simulink model "trenl"  (Simulink 8.8)
settings: Solver=ode45  StartTime=0.0  StopTime=10.0  RelTol=1e-3  EnableMultiTasking=on
values from neighbouring files (symbols this model uses):
  NP = a    [l_2.m]
  R = b    [l_2.m]
  to = randseed    [l_2.m]
  Ts = 0.001    [l_2.m]
libraries: commanapbnd3 x2
settings Model: SuppressorTable=22 serialization::archive 11 0 3 0 0 0 0 0  Creator=MichaelK  LastModifiedBy=tandav
settings DataIOCC: SaveFormat=Dataset  SignalLoggingSaveFormat=Dataset
settings DebuggingCC: UnderspecifiedInitializationDetection=Simplified  MergeDetectMultiDrivingBlocksExec=error  FcnCallInpInsideContextMsg=error  AllowSymbolicDim=off  StateNameClashWarn=none
settings HardwareCC: ProdBitPerPointer=64  ProdBitPerSizeT=64  ProdBitPerPtrDiffT=64  ProdLargestAtomicFloat=Float  ProdIntDivRoundTo=Zero  ProdEndianess=LittleEndian  ProdWordSize=64  ProdHWDeviceType=Intel->x86-64 (Windows64)
settings GRTTargetCC: GeneratePreprocessorConditionals=Use local settings  CombineOutputUpdateFcns=on  GRTInterface=off

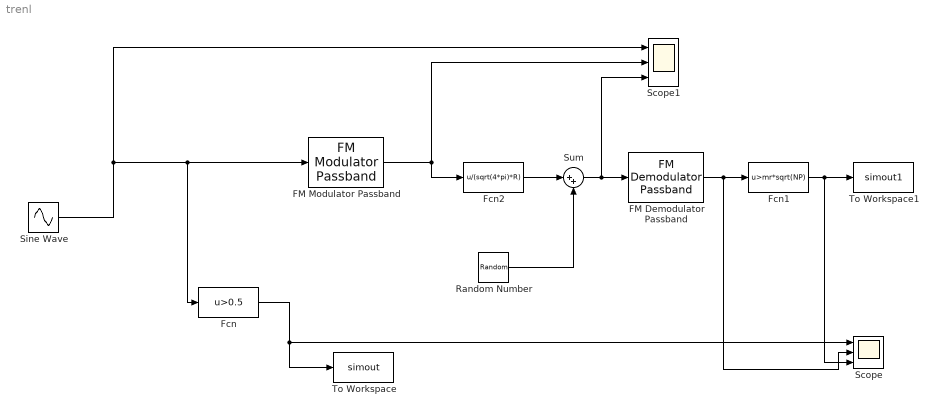
== system trenl ==
  FM Demodulator Passband : commanapbnd3/FM Demodulator Passband  Fc=500  Ph=0  Kc=50  Ho=100
  FM Modulator Passband : commanapbnd3/FM Modulator Passband  Fc=500  Ph=0  Kc=50
  Fcn : Fcn  Expr=u>0.5
  Fcn1 : Fcn  Expr=u>mr*sqrt(NP)
  Fcn2 : Fcn  Expr=u/(sqrt(4*pi)*R)
  Random Number : RandomNumber  Variance=NP  Seed=to  SampleTime=Ts
  Scope : Scope  NumInputPorts=3
  Scope1 : Scope  NumInputPorts=3
  Sine Wave : Sin  SampleTime=1
  Sum : Sum  Inputs=|++
  To Workspace : ToWorkspace  VariableName=simout  SampleTime=-1
  To Workspace1 : ToWorkspace  VariableName=simout1  SaveFormat=Timeseries  SampleTime=-1
  wires:
  Fcn/1 -> Scope/1, To Workspace/1
  FM Modulator Passband/1 -> Fcn2/1, Scope1/2
  FM Demodulator Passband/1 -> Scope/2, Fcn1/1
  Fcn1/1 -> Scope/3, To Workspace1/1
  Random Number/1 -> Sum/2
  Fcn2/1 -> Sum/1
  Sum/1 -> Scope1/3, FM Demodulator Passband/1
  Sine Wave/1 -> FM Modulator Passband/1, Fcn/1, Scope1/1
